simulink model "model_sf"  (R2016a)
settings: Solver=VariableStepAuto  StartTime=0.0  StopTime=tsim  FixedStep=0.0001  MaxStep=0.1  RelTol=1e-4
values from neighbouring files (symbols this model uses):
  alpha = 0*pi/180    (= 0)    [Chassis_ss.m]    (also in ControllerDesign.m; RunHILsim.m; RunSimulation.m; plotFrame.m = 0.196349540849)
  b = 0    [Chassis_ss.m]    (also in ControllerDesign.m; simulation.m = 0.005)
  c = 0    [Chassis_ss.m]    (also in ControllerDesign.m; simulation.m = 0.005)
  g = 9.81    [Chassis_ss.m]    (also in ControllerDesign.m; RunHILsim.m; RunSimulation.m; simulation.m = 9.82)
  I = 0.007358820323616 - M*l^2    (= 0.00237702032362)    [Chassis_ss.m]    (also in ControllerDesign.m = 0.002379687; simulation.m = 7.8125e-05)
  J = ML_J + MR_J    (= -8.16854715147e-07)    [Chassis_ss.m]    (also in ControllerDesign.m = 3.22e-06; simulation.m = 3.22e-06)
  K_dPhi = Chassis_Kc(3)    [ControllerDesign.m]    (also in ExportController.m = D(3))
  K_dTheta = Chassis_Kc(2)    [ControllerDesign.m]    (also in ExportController.m = D(2))
  K_Error = 1    [ControllerDesign.m]
  K_Theta = Chassis_Kc(1)    [ControllerDesign.m]    (also in ExportController.m = D(1))
  Kp = 2*ML_L/ML_Tau - ML_R    (= 51.7479)    [ControllerDesign.m]
  l = 95e-3    (= 0.095)    [Chassis_ss.m]    (also in ControllerDesign.m; simulation.m = 0.5)
  M = 552e-3    (= 0.552)    [Chassis_ss.m]    (also in ControllerDesign.m; simulation.m = 1)
  m = 452e-3    (= 0.452)    [Chassis_ss.m]    (also in ControllerDesign.m; simulation.m = 0.5)
  ML_Eta = 0.4    [ControllerDesign.m]
  ML_K = 0.0109    [ControllerDesign.m]
  ML_L = 0.5973    [ControllerDesign.m]
  ML_N = 30    [ControllerDesign.m]
  ML_R = 7.9821    [ControllerDesign.m]
  ML_Tm = 0.000022    (= 2.2e-05)    [ControllerDesign.m]
  r = (81.16*10^-3)/2    (= 0.04058)    [Chassis_ss.m]    (also in ControllerDesign.m = 0.041; atan2lookup.m = 1; plotFrame.m = 0.045; simulation.m = 0.045)
  T_motor = 1/1000    (= 0.001)    [ControllerDesign.m]
  T_pend = 1/100    (= 0.01)    [ControllerDesign.m]
  theta0 = 30 * pi/180    (= 0.523598775598)    [ControllerDesign.m]    (also in RunHILsim.m = 0.436332312999; RunSimulation.m = 0.0872664625997; simulation.m = 0.0872664625997)
  Vmax = 12    [ControllerDesign.m]
  vref_step_point = 1000e-3    (= 1)    [ControllerDesign.m]    (also in RunHILsim.m = 0.5; RunSimulation.m = 0.5)
libraries: cstblocks x1
settings Model: Creator=masom  LastModifiedBy=masom
settings SolverCC: ShapePreserveControl=EnableAll

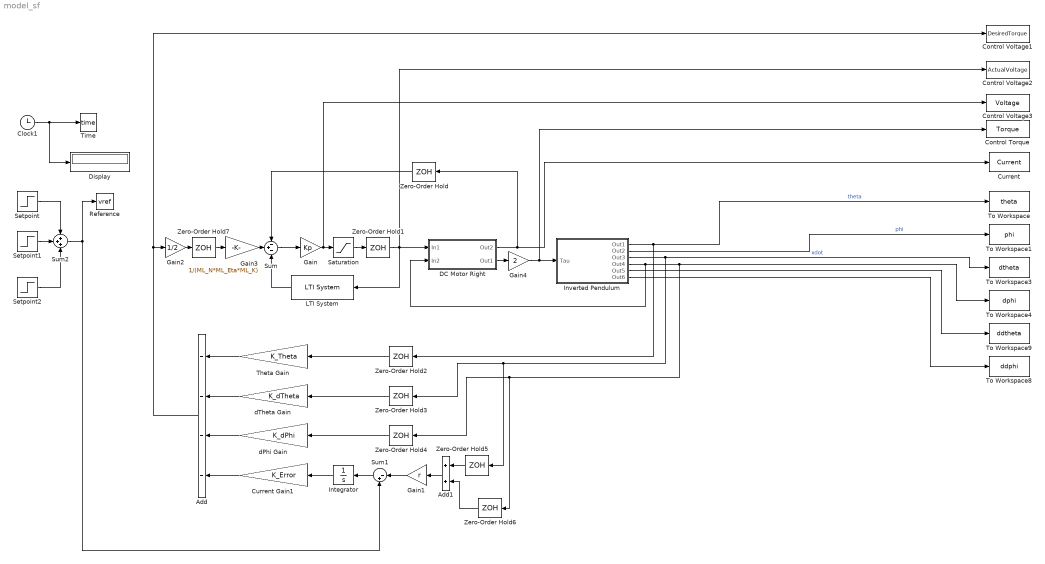
== system model_sf ==
  Add : Sum  Inputs=----
  Add1 : Sum
  Clock1 : Clock
  Control Torque : ToWorkspace  VariableName=Torque  SampleTime=-1
  Control Voltage1 : ToWorkspace  VariableName=DesiredTorque  SampleTime=-1
  Control Voltage2 : ToWorkspace  VariableName=ActualVoltage  SaveFormat=Timeseries  SampleTime=-1
  Control Voltage3 : ToWorkspace  VariableName=Voltage  SaveFormat=Timeseries  SampleTime=-1
  Current : ToWorkspace  VariableName=Current  SampleTime=-1
  Current Gain1 : Gain  Gain=K_Error
  DC Motor Right : Subsystem
  Display : Display
  Gain : Gain  Gain=Kp
  Gain1 : Gain  Gain=r
  Gain2 : Gain  Gain=1/2
  Gain3 : Gain  Gain=1/(ML_N*ML_Eta*ML_K)
  Gain4 : Gain  Gain=2
  Integrator : Integrator
  Inverted Pendulum : Subsystem
  LTI System : cstblocks/LTI System  sys=motor_ctrl  IC=[]
  Reference : ToWorkspace  VariableName=vref  SampleTime=-1
  Saturation : Saturate  UpperLimit=Vmax  LowerLimit=-Vmax
  Setpoint : Step  Time=10  After=vref_step_point  SampleTime=0
  Setpoint1 : Step  Time=11.5  After=-2*vref_step_point  SampleTime=0
  Setpoint2 : Step  Time=20  After=vref_step_point  SampleTime=0
  Sum : Sum  Inputs=-+-
  Sum1 : Sum  Inputs=|-+
  Sum2 : Sum  Inputs=+++
  Theta Gain : Gain  Gain=K_Theta
  Time : ToWorkspace  VariableName=time  SampleTime=-1
  To Workspace : ToWorkspace  VariableName=theta  SampleTime=-1
  To Workspace1 : ToWorkspace  VariableName=phi  SampleTime=-1
  To Workspace3 : ToWorkspace  VariableName=dtheta  SampleTime=-1
  To Workspace4 : ToWorkspace  VariableName=dphi  SampleTime=-1
  To Workspace8 : ToWorkspace  VariableName=ddphi  SampleTime=-1
  To Workspace9 : ToWorkspace  VariableName=ddtheta  SampleTime=-1
  Zero-Order Hold : ZeroOrderHold  SampleTime=T_motor
  Zero-Order Hold1 : ZeroOrderHold  SampleTime=T_motor
  Zero-Order Hold{2..6} (5 alike) : ZeroOrderHold  SampleTime=T_pend
  Zero-Order Hold7 : ZeroOrderHold  SampleTime=T_motor
  dPhi Gain : Gain  Gain=K_dPhi
  dTheta Gain : Gain  Gain=K_dTheta
  wires:
  Inverted Pendulum/2(Out2) -> To Workspace1/1  "phi"
  Clock1/1 -> Display/1, Time/1
  Inverted Pendulum/1(Out1) -> Zero-Order Hold2/1, To Workspace/1  "theta"
  Setpoint/1 -> Sum2/1
  Setpoint1/1 -> Sum2/2
  Sum2/1 -> Sum1/2, Reference/1
  Inverted Pendulum/3(Out3) -> Zero-Order Hold5/1, Zero-Order Hold3/1, To Workspace3/1  "xdot"
  Integrator/1 -> Current Gain1/1
  Inverted Pendulum/5(Out5) -> To Workspace9/1
  Inverted Pendulum/6(Out6) -> To Workspace8/1
  Theta Gain/1 -> Add/1
  dTheta Gain/1 -> Add/2
  dPhi Gain/1 -> Add/3
  Add1/1 -> Gain1/1
  Gain1/1 -> Sum1/1
  Sum1/1 -> Integrator/1
  Current Gain1/1 -> Add/4
  Inverted Pendulum/4(Out4) -> DC Motor Right/2(In2), Zero-Order Hold6/1, Zero-Order Hold4/1, To Workspace4/1
  DC Motor Right/2(Out1) -> Gain4/1
  Gain/1 -> Control Voltage3/1, Saturation/1
  DC Motor Right/1(Out2) -> Zero-Order Hold/1, Current/1
  Zero-Order Hold2/1 -> Theta Gain/1
  Zero-Order Hold3/1 -> dTheta Gain/1
  Zero-Order Hold4/1 -> dPhi Gain/1
  Zero-Order Hold5/1 -> Add1/1
  Zero-Order Hold6/1 -> Add1/2
  Add/1 -> Gain2/1, Control Voltage1/1
  Zero-Order Hold/1 -> Sum/1
  Sum/1 -> Gain/1
  Saturation/1 -> Zero-Order Hold1/1
  LTI System/1 -> Sum/3
  Zero-Order Hold1/1 -> DC Motor Right/1(In1), LTI System/1, Control Voltage2/1
  Zero-Order Hold7/1 -> Gain3/1
  Gain3/1 -> Sum/2
  Gain2/1 -> Zero-Order Hold7/1
  Gain4/1 -> Inverted Pendulum/1(Tau), Control Torque/1
  Setpoint2/1 -> Sum2/3

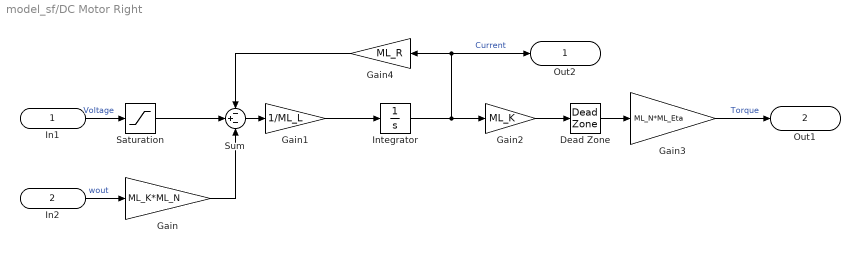
== system model_sf/DC Motor Right ==
  In1 : Inport
  In2 : Inport  Port=2
  Dead Zone : DeadZone  LowerValue=-ML_Tm  UpperValue=ML_Tm  SaturateOnIntegerOverflow=on
  Gain : Gain  Gain=ML_K*ML_N
  Gain1 : Gain  Gain=1/ML_L
  Gain2 : Gain  Gain=ML_K
  Gain3 : Gain  Gain=ML_N*ML_Eta
  Gain4 : Gain  Gain=ML_R
  Integrator : Integrator
  Saturation : Saturate  UpperLimit=Vmax  LowerLimit=-Vmax
  Sum : Sum  Inputs=-+-
  Out2 : Outport
  Out1 : Outport  Port=2
  wires:
  In1/1 -> Saturation/1  "Voltage"
  In2/1 -> Gain/1  "wout"
  Gain/1 -> Sum/3
  Sum/1 -> Gain1/1
  Gain1/1 -> Integrator/1
  Gain2/1 -> Dead Zone/1
  Dead Zone/1 -> Gain3/1
  Gain3/1 -> Out1/1  "Torque"
  Integrator/1 -> Gain4/1, Out2/1, Gain2/1  "Current"
  Gain4/1 -> Sum/1
  Saturation/1 -> Sum/2

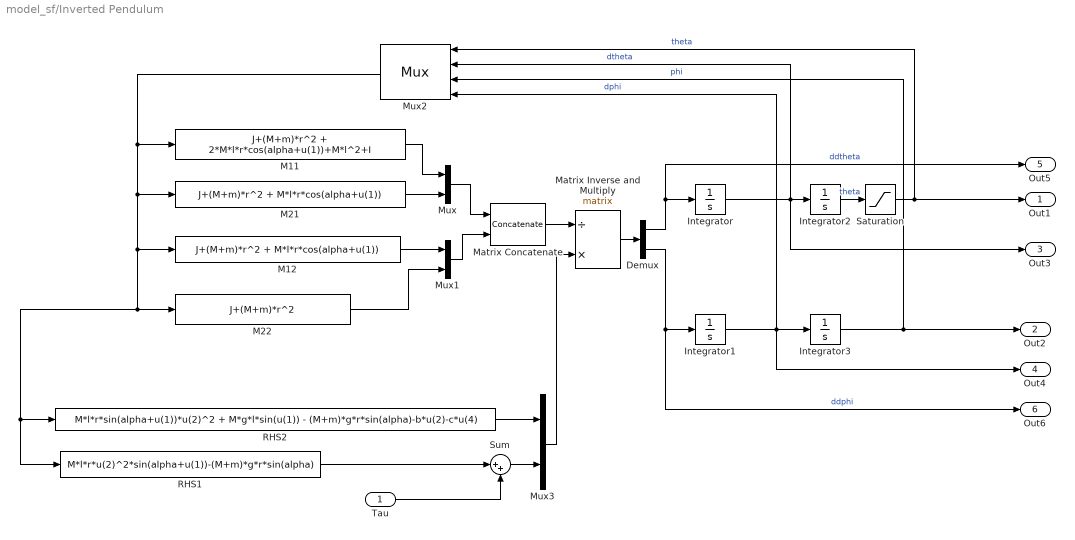
== system model_sf/Inverted Pendulum ==
  Tau : Inport
  Demux : Demux  Outputs=2
  Integrator : Integrator  ContinuousStateAttributes='dtheta'
  Integrator1 : Integrator  ContinuousStateAttributes='dphi'
  Integrator2 : Integrator  InitialCondition=theta0  ContinuousStateAttributes='theta'
  Integrator3 : Integrator  ContinuousStateAttributes='phi'
  M11 : Fcn  Expr=J+(M+m)*r^2 + 2*M*l*r*cos(alpha+u(1))+M*l^2+I
  M12 : Fcn  Expr=J+(M+m)*r^2 + M*l*r*cos(alpha+u(1))
  "M21 " : Fcn  Expr=J+(M+m)*r^2 + M*l*r*cos(alpha+u(1))
  M22 : Fcn  Expr=J+(M+m)*r^2
  Matrix Concatenate : Concatenate  Mode=Multidimensional array  ConcatenateDimension=2
  Matrix Inverse and Multiply : Product  Inputs=/*  Multiplication=Matrix(*)
  Mux : Mux  Inputs=2
  Mux1 : Mux  Inputs=2
  Mux2 : Mux
      settings: DisplayOption=signals
  Mux3 : Mux  Inputs=2
  RHS1 : Fcn  Expr=M*l*r*u(2)^2*sin(alpha+u(1))-(M+m)*g*r*sin(alpha)
  RHS2 : Fcn  Expr=M*l*r*sin(alpha+u(1))*u(2)^2 + M*g*l*sin(u(1)) - (M+m)*g*r*sin(alpha)-b*u(2)-c*u(4)
  Saturation : Saturate  UpperLimit=pi  LowerLimit=-pi
  Sum : Sum  Inputs=|++
  Out1 : Outport
  Out2 : Outport  Port=2
  Out3 : Outport  Port=3
  Out4 : Outport  Port=4
  Out5 : Outport  Port=5
  Out6 : Outport  Port=6
  wires:
  M12/1 -> Mux1/1
  Integrator1/1 -> Out4/1, Mux2/4, Integrator3/1  "dphi"
  Demux/1 -> Out5/1, Integrator/1  "ddtheta"
  Mux/1 -> Matrix Concatenate/1
  Matrix Concatenate/1 -> Matrix Inverse and Multiply/1
  Demux/2 -> Integrator1/1, Out6/1  "ddphi"
  Mux1/1 -> Matrix Concatenate/2
  RHS1/1 -> Sum/1
  Matrix Inverse and Multiply/1 -> Demux/1
  Sum/1 -> Mux3/2
  Integrator/1 -> Out3/1, Mux2/2, Integrator2/1  "dtheta"
  Integrator2/1 -> Saturation/1  "theta"
  Mux2/1 -> "M21 "/1, M22/1, RHS1/1, RHS2/1, M12/1, M11/1
  Mux3/1 -> Matrix Inverse and Multiply/2
  M11/1 -> Mux/1
  "M21 "/1 -> Mux/2
  Integrator3/1 -> Out2/1, Mux2/3  "phi"
  RHS2/1 -> Mux3/1
  Tau/1 -> Sum/2
  M22/1 -> Mux1/2
  Saturation/1 -> Out1/1, Mux2/1  "theta"
